simulink model "disc 1 sep 3 thu"  (R2026a)
settings: Solver=VariableStepAuto  MaxStep=0.02
undefined symbols (not defined in the file): c3
settings Model: Creator=tdxt  LastModifiedBy=tdxt

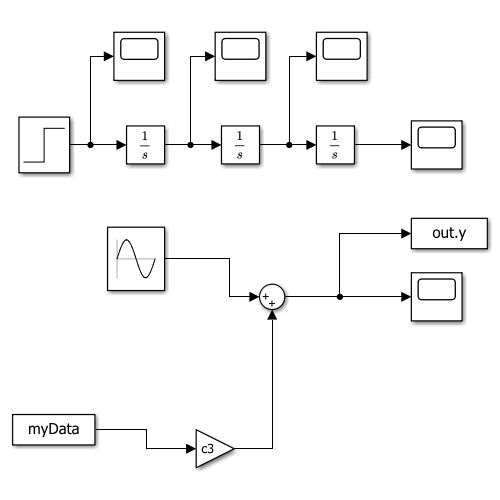
[thumbnail: Simulink's stored preview of the top-level diagram]
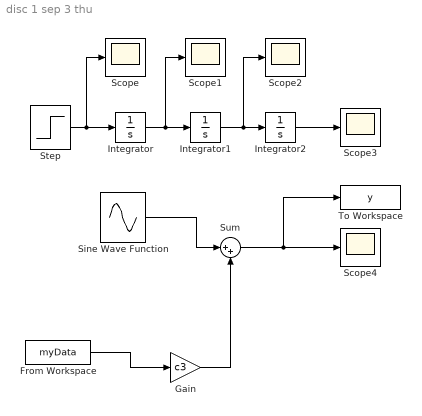
== system disc 1 sep 3 thu ==
  From Workspace : FromWorkspace  VariableName=myData
  Gain : Gain  Gain=c3
  Integrator : Integrator
  Integrator1 : Integrator
  Integrator2 : Integrator
  Scope{,1..4} (5 alike) : Scope
      Scope settings: ActiveDisplayYMinimum=-1259.2513906216086  ActiveDisplayYMaximum=1059.2291538460145
      Scope1 settings: ActiveDisplayYMinimum=-55.172226309642078  ActiveDisplayYMaximum=30.546055817132679
      Scope2 settings: ActiveDisplayYMinimum=-73.181357281596121  ActiveDisplayYMaximum=85.213170673559958  DataLoggingVariableName=ScopeData2
      Scope3 settings: ActiveDisplayYMinimum=-1516.4138338701709  ActiveDisplayYMaximum=1909.037867872556  DataLoggingVariableName=ScopeData3
      Scope4 settings: ActiveDisplayYMinimum=-4534.3682821142056  ActiveDisplayYMaximum=5402.4401886915  DataLoggingVariableName=ScopeData4
  Sine Wave Function : Sin  Amplitude=100  Frequency=10  SampleTime=0
  Step : Step  Time=2  FinalValue=FV  SampleTime=0
  Sum : Sum  Inputs=|++
  To Workspace : ToWorkspace  VariableName=y  SaveFormat=Structure With Time  SampleTime=-1
  wires:
  Gain/1 -> Sum/2
  From Workspace/1 -> Gain/1
  Sum/1 -> Scope4/1, To Workspace/1
  Sine Wave Function/1 -> Sum/1
  Step/1 -> Scope/1, Integrator/1
  Integrator/1 -> Scope1/1, Integrator1/1
  Integrator1/1 -> Scope2/1, Integrator2/1
  Integrator2/1 -> Scope3/1
